simulink model "Identification_forwardVel"  (R2020a)
settings: Solver=VariableStepAuto  StartTime=0.0  StopTime=10.0  RelTol=1e-3
values from neighbouring files (symbols this model uses):
  forwardVelocity = 1.00    (= 1)    [Part3_Identification_forVel.m]
  Krho = 1/200    (= 0.005)    [OuterLoop_forVel_rho.m]    (also in Part3_Identification_forVel.m; Part4_InnerLoop_forVel.m)
  sigrho = 20    [OuterLoop_forVel_rho.m]    (also in Part3_Identification_forVel.m; Part4_InnerLoop_forVel.m)
  Vin = 200    [Part3_Identification_forVel.m]    (also in Part3_Identification_rotVel.m)
settings Model: Creator=brett  LastModifiedBy=brett

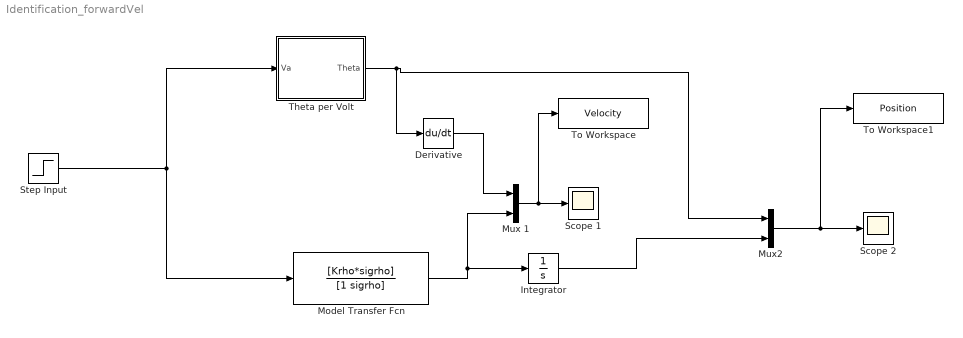
== system Identification_forwardVel ==
  Derivative : Derivative
  Integrator : Integrator
  Model Transfer Fcn : TransferFcn  Numerator=[Krho*sigrho]  Denominator=[1 sigrho]
  Mux 1 : Mux  Inputs=2
  Mux2 : Mux  Inputs=2
  Scope 1 : Scope
  Scope 2 : Scope
  Step Input : Step  After=200  SampleTime=0
  Theta per Volt : Subsystem
  To Workspace : ToWorkspace  VariableName=Velocity  SaveFormat=Timeseries  SampleTime=-1
  To Workspace1 : ToWorkspace  VariableName=Position  SaveFormat=Timeseries  SampleTime=-1
  wires:
  Mux 1/1 -> To Workspace/1, Scope 1/1
  Mux2/1 -> To Workspace1/1, Scope 2/1
  Derivative/1 -> Mux 1/1
  Model Transfer Fcn/1 -> Mux 1/2, Integrator/1
  Integrator/1 -> Mux2/2
  Theta per Volt/1(Theta) -> Derivative/1, Mux2/1
  Step Input/1 -> Model Transfer Fcn/1, Theta per Volt/1(Va)

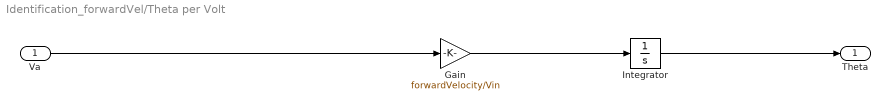
== system Identification_forwardVel/Theta per Volt ==
  Va : Inport
  Gain : Gain  Gain=forwardVelocity/Vin
  Integrator : Integrator
  Theta : Outport
  wires:
  Va/1 -> Gain/1
  Gain/1 -> Integrator/1
  Integrator/1 -> Theta/1
